simulink model "OEWIM_SinePWM"  (R2023b)
settings: Solver=VariableStepAuto  StartTime=0.0  StopTime=10.0  RelTol=1e-3
InitFcn:
  | P=4
undefined symbols (not defined in the file): DiscIntNeverNeededParam
libraries: spsIGBTDiodeLib x12, spsDCVoltageSourceLib x2, spsAsynchronousMachineSIUnitsLib x1
settings Model: Creator=HP  LastModifiedBy=HP

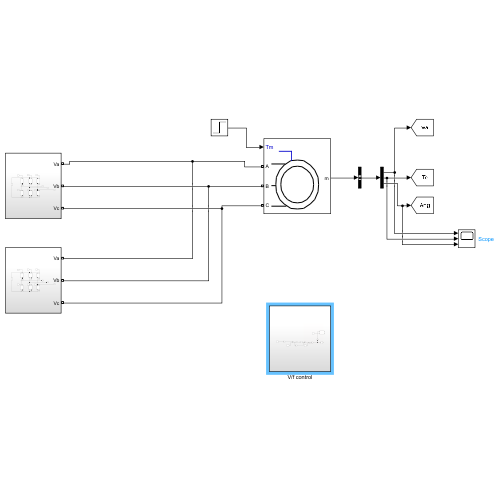
[thumbnail: Simulink's stored preview of the top-level diagram]
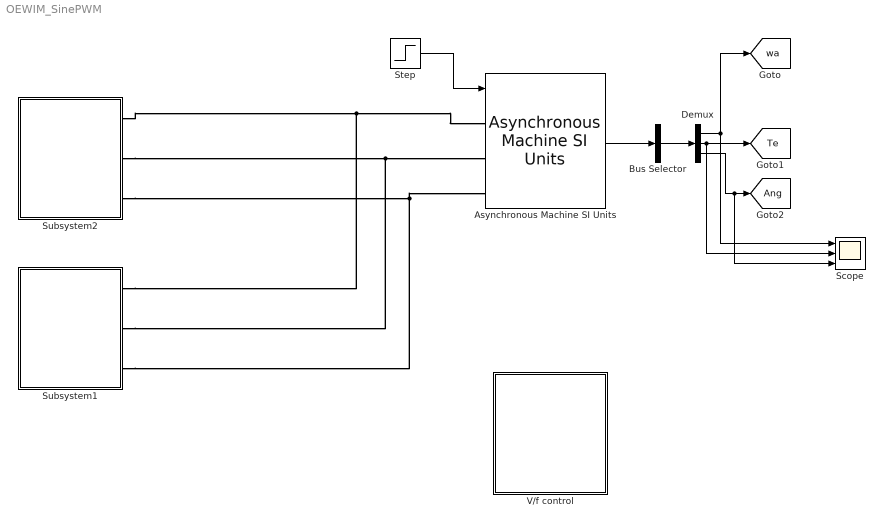
== system OEWIM_SinePWM ==
  Asynchronous Machine SI Units : spsAsynchronousMachineSIUnitsLib/Asynchronous Machine SI Units  RotorType=Squirrel-cage  PresetModel=No  MechanicalLoad=Torque Tm  ShowDetailedParameters=on  ReferenceFrame=Rotor  Units=SI  MeasurementBus=off  NominalParameters=[1.845e+04 400 50]  VoltageRatio=1  Stator=[0.5968 0.0003495]  Rotor=[0.6258 0.005473]  Cage1=[0.4155 0.002066]  Cage2=[0.4168 0.0003495]  Lm=0.0354  Mechanical=[0.05 0.005879 2]  PolePairs=2  InitialConditions=[0 0 0 0 0 0 0 0]  SimulateSaturation=off  Saturation=[14.03593122, 27.81365428, 53.79336849, 72.68890987, 97.98006896, 148.6815601, 215.7428561, 302.9841135, 428.7778367 ; 230, 322, 414, 460, 506, 552, 598, 644, 690]  LoadFlowParameters=1492000  TsPowergui=0  TsBlock=-1  IterativeModel=Trapezoidal non iterative  IterativeDiscreteModel=Trapezoidal non iterative  Pmec=1.492e+006
  Bus Selector : BusSelector  OutputSignals=Mechanical.Rotor speed (wm),Mechanical.Electromagnetic torque Te (N*m),Mechanical.Rotor angle thetam (rad)  OutputAsBus=on
  Demux : Demux  Outputs=3
  Scope : Scope  NumInputPorts=3
  Step : Step  SampleTime=0
  Subsystem1 : Subsystem
  Subsystem2 : Subsystem
  V/f control : Subsystem
  tag scope: Ang=global, Te=global, wa=global
  wires:
  Step/1 -> Asynchronous Machine SI Units/1
  Asynchronous Machine SI Units/1 -> Bus Selector/1
  Bus Selector/1 -> Demux/1
  Demux/1 -> [wa], Scope/1
  Demux/2 -> Scope/2, [Te]
  Demux/3 -> Scope/3, [Ang]
  connections:
  Subsystem2/RConn1 -- Subsystem1/RConn1 -- Asynchronous Machine SI Units/LConn1
  Subsystem2/RConn2 -- Subsystem1/RConn2 -- Asynchronous Machine SI Units/LConn2
  Subsystem2/RConn3 -- Asynchronous Machine SI Units/LConn3 -- Subsystem1/RConn3

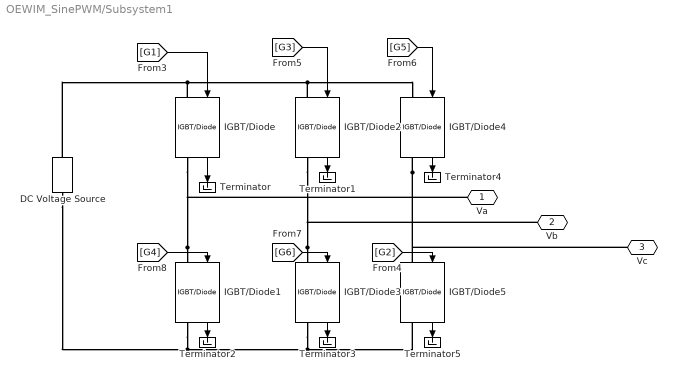
== system OEWIM_SinePWM/Subsystem1 ==
  DC Voltage Source : spsDCVoltageSourceLib/DC Voltage Source  Amplitude=162  Measurements=None
  IGBT/Diode{,1..5} (6 alike) : spsIGBTDiodeLib/IGBT//Diode  Ron=1e-3  Rs=1e5  Cs=inf  Measurements=on
  Terminator{,1..5} (6 alike) : Terminator
  Va : PMIOPort  Side=Right
  Vb : PMIOPort  Port=2  Side=Right
  Vc : PMIOPort  Port=3  Side=Right
  wires:
  [G6] -> IGBT/Diode3/1
  IGBT/Diode5/1 -> Terminator5/1
  IGBT/Diode2/1 -> Terminator1/1
  [G5] -> IGBT/Diode4/1
  [G3] -> IGBT/Diode2/1
  IGBT/Diode/1 -> Terminator/1
  [G4] -> IGBT/Diode1/1
  IGBT/Diode1/1 -> Terminator2/1
  [G1] -> IGBT/Diode/1
  [G2] -> IGBT/Diode5/1
  IGBT/Diode4/1 -> Terminator4/1
  IGBT/Diode3/1 -> Terminator3/1
  connections:
  IGBT/Diode3/LConn1 -- Vb/RConn1 -- IGBT/Diode2/RConn1
  IGBT/Diode1/LConn1 -- Va/RConn1 -- IGBT/Diode/RConn1
  IGBT/Diode4/RConn1 -- IGBT/Diode5/LConn1 -- Vc/RConn1
  DC Voltage Source/RConn1 -- IGBT/Diode/LConn1 -- IGBT/Diode2/LConn1 -- IGBT/Diode4/LConn1
  DC Voltage Source/LConn1 -- IGBT/Diode1/RConn1 -- IGBT/Diode5/RConn1 -- IGBT/Diode3/RConn1

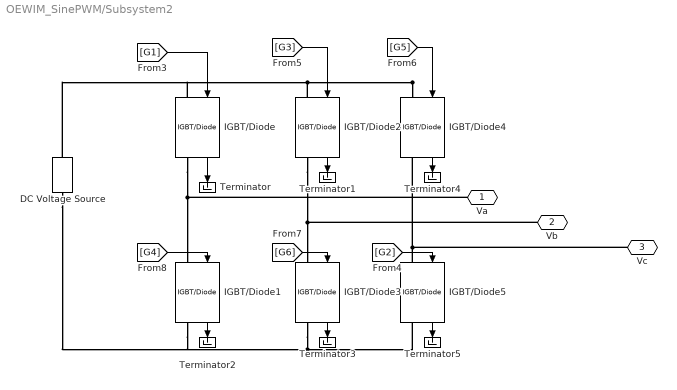
== system OEWIM_SinePWM/Subsystem2 ==
  DC Voltage Source : spsDCVoltageSourceLib/DC Voltage Source  Amplitude=162  Measurements=None
  IGBT/Diode{,1..5} (6 alike) : spsIGBTDiodeLib/IGBT//Diode  Ron=1e-3  Rs=1e5  Cs=inf  Measurements=on
  Terminator{,1..5} (6 alike) : Terminator
  Va : PMIOPort  Side=Right
  Vb : PMIOPort  Port=2  Side=Right
  Vc : PMIOPort  Port=3  Side=Right
  wires:
  IGBT/Diode3/1 -> Terminator3/1
  IGBT/Diode4/1 -> Terminator4/1
  [G2] -> IGBT/Diode5/1
  [G1] -> IGBT/Diode/1
  IGBT/Diode1/1 -> Terminator2/1
  [G4] -> IGBT/Diode1/1
  IGBT/Diode/1 -> Terminator/1
  [G3] -> IGBT/Diode2/1
  [G5] -> IGBT/Diode4/1
  IGBT/Diode2/1 -> Terminator1/1
  IGBT/Diode5/1 -> Terminator5/1
  [G6] -> IGBT/Diode3/1
  connections:
  IGBT/Diode3/RConn1 -- DC Voltage Source/LConn1 -- IGBT/Diode1/RConn1 -- IGBT/Diode5/RConn1
  IGBT/Diode4/LConn1 -- DC Voltage Source/RConn1 -- IGBT/Diode/LConn1 -- IGBT/Diode2/LConn1
  Vc/RConn1 -- IGBT/Diode5/LConn1 -- IGBT/Diode4/RConn1
  IGBT/Diode/RConn1 -- IGBT/Diode1/LConn1 -- Va/RConn1
  IGBT/Diode2/RConn1 -- Vb/RConn1 -- IGBT/Diode3/LConn1

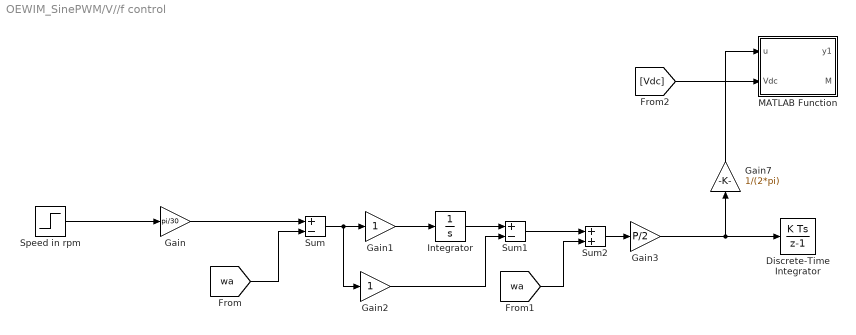
== system OEWIM_SinePWM/V//f control ==
  Discrete-Time Integrator : DiscreteIntegrator  gainval=1  SampleTime=-1  ICPrevOutput=DiscIntNeverNeededParam  ICPrevScaledInput=DiscIntNeverNeededParam
  Gain : Gain  Gain=pi/30
  Gain1 : Gain
  Gain2 : Gain
  Gain3 : Gain  Gain=P/2
  Gain7 : Gain  Gain=1/(2*pi)
  Integrator : Integrator
  MATLAB Function : MATLAB Function  TreatAsAtomicUnit=on
  Speed in rpm : Step  SampleTime=0
  Sum : Sum  Inputs=+-
  Sum1 : Sum  Inputs=+-
  Sum2 : Sum
  wires:
  Speed in rpm/1 -> Gain/1
  [wa] -> Sum/2
  Gain/1 -> Sum/1
  Sum/1 -> Gain2/1, Gain1/1
  Gain1/1 -> Integrator/1
  Integrator/1 -> Sum1/1
  Gain2/1 -> Sum1/2
  Sum1/1 -> Sum2/1
  [wa] -> Sum2/2
  Sum2/1 -> Gain3/1
  Gain3/1 -> Discrete-Time Integrator/1, Gain7/1
  Gain7/1 -> MATLAB Function/1(u)
  [Vdc] -> MATLAB Function/2(Vdc)

== matlab function OEWIM_SinePWM/V//f control/MATLAB Function ==
  data: u input; y1 output; Vdc input; M output
function [y1, M] = fcn(u,Vdc)


if u<5
    y1 = 23/sqrt(3);
    
elseif (u>=5) && (u<=50)
    y1 = ((230/(sqrt(3))*u)/50);
    
else
    y1=230/sqrt(3);
end

M =(sqrt(2)*y1*pi)/(2*Vdc);
end
